simulink model "MRAC"  (R2022b)
settings: Solver=VariableStepAuto  StartTime=0.0  StopTime=10.0  RelTol=1e-3
settings Model: Creator=rajen  LastModifiedBy=laksh

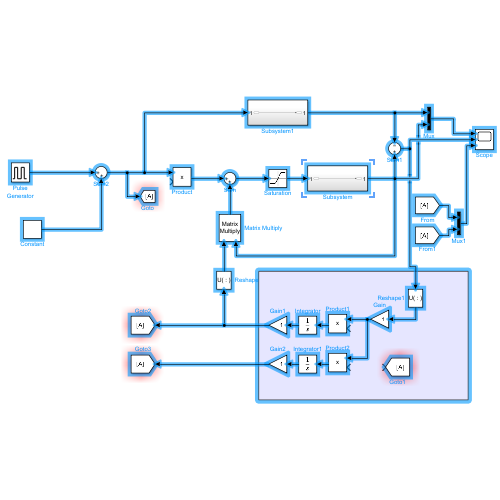
[thumbnail: Simulink's stored preview of the top-level diagram]
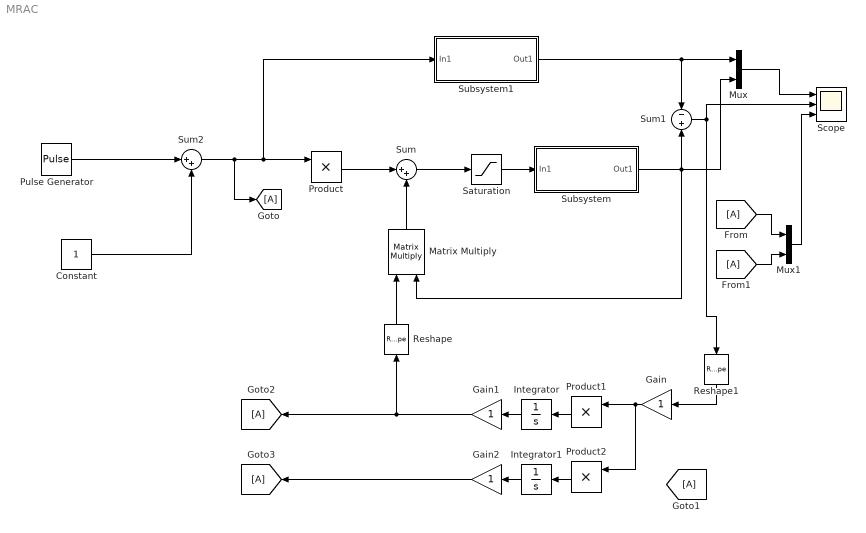
== system MRAC ==
  Constant : Constant
  From : From
  From1 : From
  Gain : Gain
  Gain1 : Gain
  Gain2 : Gain
  Goto{,1..3} (4 alike) : Goto
  Integrator : Integrator
  Integrator1 : Integrator
  Matrix Multiply : Product  Multiplication=Matrix(*)
  Mux : Mux  Inputs=2
  Mux1 : Mux  Inputs=2
  Product : Product
  Product1 : Product
  Product2 : Product
  Pulse Generator : DiscretePulseGenerator  PulseType=Time based  Period=10  PulseWidth=5
  Reshape : Reshape
  Reshape1 : Reshape
  Saturation : Saturate
  Scope : Scope  NumInputPorts=3
  Subsystem : Subsystem
  Subsystem1 : Subsystem
  Sum : Sum  Inputs=|++
  Sum1 : Sum  Inputs=-|+
  Sum2 : Sum  Inputs=|++
  wires:
  Product/1 -> Sum/1
  Sum/1 -> Saturation/1
  Saturation/1 -> Subsystem/1(In1)
  From/1 -> Mux1/1
  From1/1 -> Mux1/2
  Mux/1 -> Scope/1
  Subsystem/1(Out1) -> Mux/2, Matrix Multiply/2, Sum1/2
  Matrix Multiply/1 -> Sum/2
  Reshape/1 -> Matrix Multiply/1
  Sum2/1 -> Goto/1, Subsystem1/1(In1), Product/1
  Pulse Generator/1 -> Sum2/1
  Constant/1 -> Sum2/2
  Reshape1/1 -> Gain/1
  Product1/1 -> Integrator/1
  Product2/1 -> Integrator1/1
  Gain/1 -> Product1/1, Product2/1
  Integrator/1 -> Gain1/1
  Integrator1/1 -> Gain2/1
  Gain1/1 -> Reshape/1, Goto2/1
  Gain2/1 -> Goto3/1
  Subsystem1/1(Out1) -> Sum1/1, Mux/1
  Sum1/1 -> Reshape1/1, Scope/2
  Mux1/1 -> Scope/3

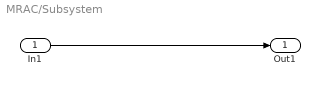
== system MRAC/Subsystem ==
  In1 : Inport
  Out1 : Outport
  wires:
  In1/1 -> Out1/1

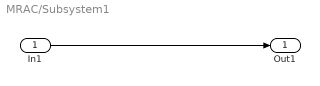
== system MRAC/Subsystem1 ==
  In1 : Inport
  Out1 : Outport
  wires:
  In1/1 -> Out1/1
